simulink model "P_2_3_parabolic_error"  (R2021a)
settings: Solver=VariableStepAuto  StartTime=0.0  StopTime=25  RelTol=1e-3
settings Model: Creator=alamg  LastModifiedBy=alamg

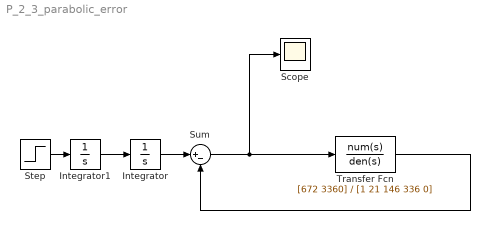
== system P_2_3_parabolic_error ==
  Integrator : Integrator
  Integrator1 : Integrator
  Scope : Scope
  Step : Step  SampleTime=0
  Sum : Sum  Inputs=|+-
  Transfer Fcn : TransferFcn  Numerator=[672 3360]  Denominator=[1 21 146 336 0]
  wires:
  Sum/1 -> Transfer Fcn/1, Scope/1
  Transfer Fcn/1 -> Sum/2
  Integrator1/1 -> Integrator/1
  Integrator/1 -> Sum/1
  Step/1 -> Integrator1/1
